simulink model "Purdue_Sim"  (R2018b)
settings: Solver=VariableStepAuto  StartTime=0.0  StopTime=300  FixedStep=0.0001  RelTol=1e-7
values from neighbouring files (symbols this model uses):
  alpha_data = load('alpha_data.csv')    [One_Run.m]    (also in Test_Runs_Arthur_Function.m; eqns_motion_script.m; eqns_motion_script_439.m)
  AR = De^2/Dt^2    (= 7.35623218146)    [One_Run.m]    (also in Test_Runs_Arthur_Function.m; engineMass.m = engine.output.eql.aeat(3); eqns_motion_script_439.m = 7.52170654272)
  At = pi*Dt^2/4    (= 7.87496924005)    [One_Run.m]    (also in Test_Runs_Arthur_Function.m; engineMass.m = cstar*mdot/(Pc*g); eqns_motion_script_439.m = 7.53210209316)
  burn_time = (200000+Impulse_Savings)/Thrust    (= 39.2156862745)    [One_Run.m]    (also in Purdue_Setup.m = 40; Setup.m = 42; Test_Runs.m = 40; Test_Runs_Arthur_Function.m = 42.7553241067)
  Cd_data = load('cd_M.csv')    [One_Run.m]    (also in Test_Runs_Arthur_Function.m; eqns_motion_script.m; eqns_motion_script_439.m)
  Cn_data = load('cl_M_a.csv')    [One_Run.m]    (also in Test_Runs_Arthur_Function.m; eqns_motion_script.m; eqns_motion_script_439.m)
  Cp_data = load('cp_M_a.csv')    [One_Run.m]    (also in Test_Runs_Arthur_Function.m; eqns_motion_script.m; eqns_motion_script_439.m)
  De = 8.5883    [One_Run.m]    (also in Test_Runs_Arthur_Function.m; engineMass.m = sqrt(4*Ae/pi); eqns_motion_script_439.m = 8.4932)
  diameter_ft = diameter/12    (= 1.5)    [One_Run.m]    (also in Purdue_Setup.m; Setup.m = 0.535416666667; Test_Runs.m; Test_Runs_Arthur_Function.m)
  dry_mass_slugs = dry_mass / 32.2    (= 16.4109852637)    [One_Run.m]    (also in Purdue_Setup.m = 12.4223602484; Setup.m = 1.28260869565; Test_Runs.m = dry_mass / 32.2; Test_Runs_Arthur_Function.m = dry_mass / 32.2)
  initial_height = 4595    [One_Run.m]    (also in Purdue_Setup.m = 4600; Setup.m = 0; Test_Runs.m = 0; Test_Runs_Arthur_Function.m)
  latitude = 32.9861    [One_Run.m]    (also in Test_Runs_Arthur_Function.m)
  longitude = -106.9717    [One_Run.m]    (also in Test_Runs_Arthur_Function.m)
  M_data = load('M_data.csv')    [One_Run.m]    (also in Test_Runs_Arthur_Function.m; eqns_motion_script.m; eqns_motion_script_439.m)
  m_dot_slugs = m_dot / 32.2    (= 0.725155279503)    [One_Run.m]    (also in Purdue_Setup.m = -0.621118012422; Setup.m = 0.0567139899438; Test_Runs.m = -0.621118012422; Test_Runs_Arthur_Function.m = -0.62217941157)
  mass_inert = 523.36 + margin    (= 523.36)    [One_Run.m]    (also in Setup.m = 41.3; Test_Runs.m = mass_engine + mass_pump + tank(1).mass +tank(2).mass + mass_; Test_Runs_Arthur_Function.m = mass_engine + mass_pump + tank(1).mass +tank(2).mass + inter)
  Pc = 450    [One_Run.m]    (also in Test_Runs_Arthur_Function.m; eqns_motion_script_439.m)
  Pe = 10    [One_Run.m]    (also in Test_Runs.m = pressure_integral(end)/burn_time; Test_Runs_Arthur_Function.m; eqns_motion_script_439.m)
  rocket_length = 24    [One_Run.m]    (also in Setup.m; Test_Runs.m; Test_Runs_Arthur_Function.m)
  Throttle_end_time = 35    [One_Run.m]    (also in Setup.m; Test_Runs.m = 0; Test_Runs_Arthur_Function.m = 0)
  Throttle_start_time = 15    [One_Run.m]    (also in Setup.m; Test_Runs.m = 0; Test_Runs_Arthur_Function.m = 0)
  Throttled_m_dot = m_dot_slugs*(1 - throttle)    (= 0.725155279503)    [One_Run.m]    (also in Setup.m = 0.0567139899438; Test_Runs.m = -0.621118012422; Test_Runs_Arthur_Function.m = -0.62217941157)
  Thrust = 5100    [One_Run.m]    (also in Purdue_Setup.m = 5000; Setup.m = 800; Test_Runs.m = 5000; Test_Runs_Arthur_Function.m = 4677.78)
  wet_mass_slugs = wet_mass / 32.2    (= 44.848447205)    [One_Run.m]    (also in Purdue_Setup.m = 37.2670807453; Setup.m = 3.66459627329; Test_Runs.m = wet_mass / 32.2; Test_Runs_Arthur_Function.m = wet_mass / 32.2)
libraries: vrlib x8, aerolibconvert2 x5, aerolibasang x3, simulink_extras x3, aerolibutil x2, simulink x2, aerolibanimutils x2, shared6dof x1, sharedutil x1, aerolibadyn x1, aerolibatmos2 x1, aerolibtransform2 x1
settings Model: Creator=jbartkie  LastModifiedBy=bartk
settings DataIOCC: ExternalInput=getinputstruct(op_snapshot1)  InitialState=getstatestruct(op_snapshot1)
settings DebuggingCC: LibraryContextMissingDiagnostic=none
settings SFSimCC: SimUseLocalCustomCode=off
settings RTWCC: RTWUseLocalCustomCode=off

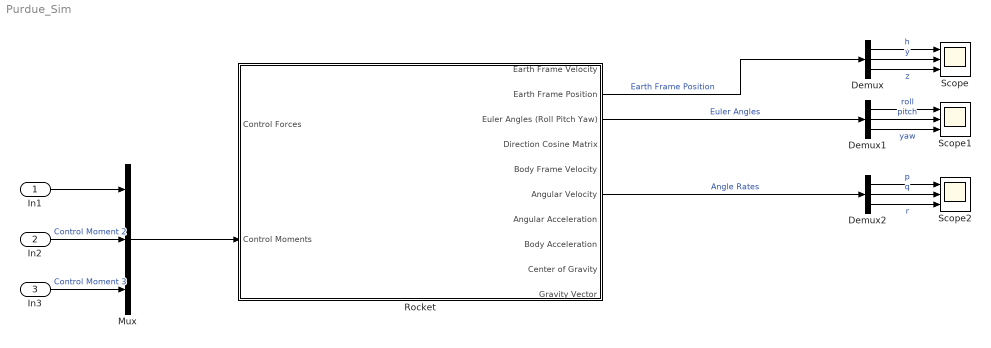
== system Purdue_Sim ==
  In1 : Inport
  In2 : Inport  Port=2
  In3 : Inport  Port=3
  Demux : Demux  Outputs=3
  Demux1 : Demux  Outputs=3
  Demux2 : Demux  Outputs=3
  Mux : Mux  Inputs=3
  Rocket : Subsystem
  Scope : Scope  NumInputPorts=3
  Scope1 : Scope  NumInputPorts=3
  Scope2 : Scope  NumInputPorts=3
  wires:
  Mux/1 -> Rocket/2(Control Moments)
  In2/1 -> Mux/2  "Control Moment 2"
  In3/1 -> Mux/3  "Control Moment 3"
  Rocket/6(Angular Velocity) -> Demux2/1  "Angle Rates"
  Rocket/3(Euler Angles (Roll Pitch Yaw)) -> Demux1/1  "Euler Angles"
  Rocket/2(Earth Frame Position) -> Demux/1  "Earth Frame Position"
  Demux/1 -> Scope/1  "h"
  Demux/2 -> Scope/2  "y"
  Demux/3 -> Scope/3  "z"
  Demux1/1 -> Scope1/1  "roll"
  Demux1/2 -> Scope1/2  "pitch"
  Demux1/3 -> Scope1/3  "yaw"
  Demux2/1 -> Scope2/1  "p"
  Demux2/2 -> Scope2/2  "q"
  Demux2/3 -> Scope2/3  "r"
  In1/1 -> Mux/1

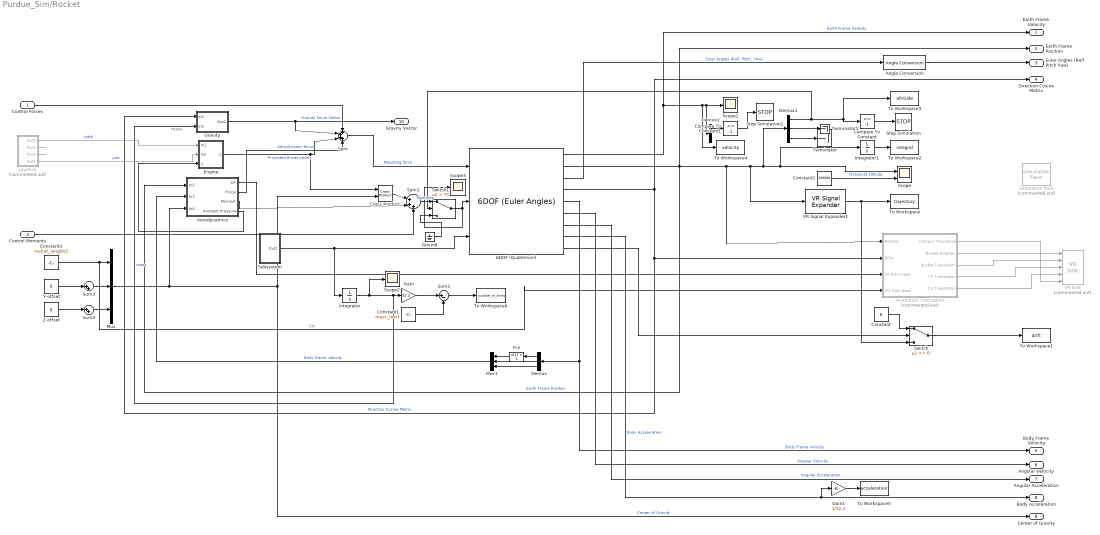
== system Purdue_Sim/Rocket ==
  note: mass
  Control Forces : Inport
  Control Moments : Inport  Port=2
  6DOF (Quaternion) : shared6dof/6DOF (Euler Angles)  units=English (Velocity in ft/s)  mtype=Simple Variable  rep=Quaternion  xme_0=[initial_height 0 0]  Vm_0=[0 0 0]  eul_0=[0 0*pi/180 0]  pm_0=[0 0 0]  mass_0=wet_mass_slugs  mass_e=dry_mass_slugs  mass_f=wet_mass_slugs  inertia=eye(3)  inertia_e=I_wet  inertia_f=I_dry  k_quat=1.0  vre_flag=off  abi_flag=off  aMode=0  xme_statename=''  Vm_statename=''  eul_statename=''  quat_statename=''  pm_statename=''  mass_statename=''
      settings: SourceProductBaseCode=AE
  "Aerodynamics " : Subsystem
  Angle Conversion : aerolibconvert2/Angle Conversion  IU=rad  OU=deg
  Animation Translation : Subsystem  Commented=on
  Compare To Constant : simulink/Logic and Bit Operations/Compare To Constant  relop=<=  const=-1  OutDataTypeStr=boolean
  Compare To Constant1 : simulink/Logic and Bit Operations/Compare To Constant  relop=<=  const=-1  OutDataTypeStr=boolean
  Constant : Constant  Value=0
  Constant1 : Constant  Value=mass_inert
  Constant2 : Constant  Value=328084
  Constant3 : Constant  Value=rocket_length/2
  Cross Product : vrlib/Utilities/Cross Product
      settings: SourceProductBaseCode=VR
  Demux : Demux  Outputs=3
  Demux1 : Demux  Outputs=3
  Demux2 : Demux  Outputs=3
  "Engine " : Subsystem
  Fcn : Fcn  Expr=u(1) + 1
  Gain : Gain  Gain=32.2
  Gain1 : Gain  Gain=1/32.2
  Gravity : Subsystem
  Ground : Ground
  Integrator : Integrator  InitialCondition=wet_mass_slugs  LimitOutput=on  LowerSaturationLimit=dry_mass_slugs
  Integrator1 : Integrator
  Joystick : Subsystem  Commented=on
  Mux : Mux  Inputs=3
  Mux1 : Mux  Inputs=3
  Scope : Scope  NumInputPorts=2
  Scope1 : Scope
  Scope2 : Scope
  Scope3 : Scope
  Simulation Pace : aerolibanimutils/Simulation Pace  Commented=on  SimulationPace=1  SleepMode=MATLAB Thread  OutputPaceError=off  SampleTime=1/30
  Stop Simulation : Stop
  Stop Simulation1 : Stop
  Subsystem : Subsystem
  Sum : Sum  Inputs=++++
  Sum1 : Sum  Inputs=|+++
  Sum2 : Sum  Inputs=|+-
  Sum3 : Sum  Inputs=|++
  Sum4 : Sum  Inputs=|++
  Switch : Switch
  Switch1 : Switch  Criteria=u2 > Threshold  Threshold=75
  Terminator : Terminator
  Terminator1 : Terminator
  To Workspace : ToWorkspace  VariableName=trajectory  SampleTime=-1
  To Workspace1 : ToWorkspace  VariableName=drift  SampleTime=-1
  To Workspace2 : ToWorkspace  VariableName=integral  SampleTime=-1
  To Workspace3 : ToWorkspace  VariableName=altitude  SampleTime=-1
  To Workspace4 : ToWorkspace  VariableName=velocity  SampleTime=-1
  To Workspace5 : ToWorkspace  VariableName=acceleration  SampleTime=-1
  To Workspace6 : ToWorkspace  VariableName=oxidizer_m_array  SampleTime=-1
  VR Signal Expander1 : vrlib/VR Signal Expander  outwidth=3  outidx=[3 2 1]
      settings: SourceProductName=Simulink 3D Animation  SourceProductBaseCode=VR
  VR Sink : vrlib/VR Sink  Commented=on  InstantiateOnLoad=on  SampleTime=0.1  ViewEnable=on  RemoteChange=off  RemoteView=off  FieldsWritten=Rocket.rotation.4.1.1.double#Rocket.translation.3.1.1.double#CP.translation.3.1.1.double#CG.translation.3.1.1.double#Camera.position.3.1.1.double  WorldFileName=liftoff.WRL  AutoView=off  VideoDimensions=[]  AllowVariableSize=off
      settings: SourceProductBaseCode=VR
  Y-offset : Constant  Value=0
  Z-offset : Constant  Value=0
  Earth Frame Velocity : Outport
  Earth Frame Position : Outport  Port=2
  Euler Angles (Roll Pitch Yaw) : Outport  Port=3
  Direction Cosine Matrix : Outport  Port=4
  Body Frame Velocity : Outport  Port=5
  Angular Velocity : Outport  Port=6
  Angular Acceleration : Outport  Port=7
  Body Acceleration : Outport  Port=8
  Center of Gravity : Outport  Port=9
  Gravity Vector : Outport  Port=10
  wires:
  Demux/3 -> Mux1/3
  6DOF (Quaternion)/4 -> Gravity/1(In1), Animation Translation/2(DCM), Direction Cosine Matrix/1  "Direction Cosine Matrix"
  6DOF (Quaternion)/2 -> VR Signal Expander1/1, Demux1/1, Integrator1/1, Scope/1, Animation Translation/1(Position), "Aerodynamics "/1(In2), Earth Frame Position/1  "Earth Frame Position"
  6DOF (Quaternion)/1 -> Earth Frame Velocity/1, To Workspace4/1, Demux2/1, Scope1/1  "Earth Frame Velocity"
  6DOF (Quaternion)/3 -> Angle Conversion/1  "Euler Angles (Roll, Pitch, YAw)"
  6DOF (Quaternion)/7 -> Angular Acceleration/1  "Angular Acceleration"
  6DOF (Quaternion)/8 -> Gain1/1, Body Acceleration/1  "Body Acceleration"
  Mux/1 -> Cross Product/2, Center of Gravity/1, "Aerodynamics "/3(In4)  "Center of Gravity"
  6DOF (Quaternion)/6 -> Angular Velocity/1  "Angular Velocity"
  Cross Product/1 -> Sum1/1
  Gravity/1(Out1) -> Gravity Vector/1, Sum/2  "Gravity Force Vector"
  6DOF (Quaternion)/5 -> Demux/1, Body Frame Velocity/1  "Body Frame Velocity"
  Control Moments/1 -> Sum1/3
  Control Forces/1 -> Sum/1
  Integrator/1 -> Scope2/1, Gravity/2(In2), Gain/1  "mass"
  Sum/1 -> 6DOF (Quaternion)/1  "Resulting force"
  Joystick/1(Out1) -> "Engine "/1(In1)  "pitch"
  "Engine "/1(Out1) -> Cross Product/1, Sum/3  "Projected thrust vector"
  Demux1/3 -> Terminator/1
  Joystick/4(Out4) -> "Engine "/2(In2)  "yaw"
  Switch/1 -> To Workspace1/1
  Demux/2 -> Mux1/2
  Demux/1 -> Fcn/1
  Fcn/1 -> Mux1/1
  Mux1/1 -> "Aerodynamics "/2(In3)  "Body frame velocity"
  VR Signal Expander1/1 -> Switch/3, To Workspace/1
  "Aerodynamics "/1(CP) -> Animation Translation/3(CP from base)
  Constant/1 -> Switch/1
  Joystick/2(Out2) -> ?
  Compare To Constant/1 -> Stop Simulation/1
  Integrator1/1 -> To Workspace2/1
  Joystick/3(Out3) -> ?
  Demux1/2 -> Terminator1/1
  Demux1/1 -> Switch1/2, Compare To Constant/1, To Workspace3/1
  6DOF (Quaternion)/9 -> Switch/2
  Constant3/1 -> Mux/1, Animation Translation/4(CG from base)  "CG"
  Animation Translation/2(Rocket Rotation) -> VR Sink/1
  Animation Translation/3(Rocket Translation) -> VR Sink/2
  Animation Translation/4(CP Translation) -> VR Sink/3
  Animation Translation/5(CG Translation) -> VR Sink/4
  Animation Translation/1(Camera Translation) -> VR Sink/5
  Constant2/1 -> Scope/2  "threshold altitude"
  Angle Conversion/1 -> Euler Angles (Roll Pitch Yaw)/1
  "Aerodynamics "/3(Moment) -> Sum1/2
  "Aerodynamics "/2(Force) -> Sum/4  "Aerodynamic force"
  Constant1/1 -> Sum2/2
  Gain/1 -> Sum2/1
  Sum2/1 -> To Workspace6/1
  Compare To Constant1/1 -> Stop Simulation1/1
  Y-offset/1 -> Sum3/1
  Sum3/1 -> Mux/2
  Z-offset/1 -> Sum4/1
  Sum4/1 -> Mux/3
  Demux2/1 -> Compare To Constant1/1
  Subsystem/1(Out1) -> 6DOF (Quaternion)/3, Integrator/1
  Gain1/1 -> To Workspace5/1
  "Aerodynamics "/4(Ambient Pressure) -> "Engine "/3(Ambient Pressure)
  Sum1/1 -> Switch1/1  "Moments"
  Switch1/1 -> 6DOF (Quaternion)/2, Scope3/1
  Ground/1 -> Switch1/3

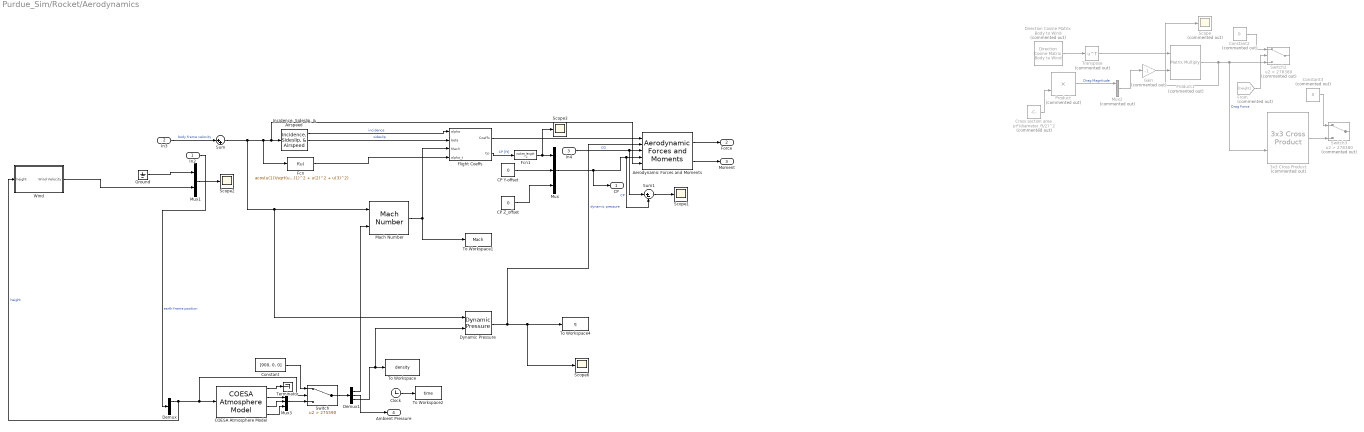
== system Purdue_Sim/Rocket/Aerodynamics  ==
  In2 : Inport
  In3 : Inport  Port=2
  In4 : Inport  Port=3
  3x3 Cross Product : sharedutil/3x3 Cross Product  Commented=on  aMode=aMode
      settings: SourceProductBaseCode=AE
  "Aerodynamic Forces and Moments " : aerolibadyn/Aerodynamic Forces and Moments   inputAxes=Wind  outputForceAxes=Body  outputMomentAxes=Body  S=S  b=diameter_ft  cbar=rocket_length
      settings: SourceProductName=Aerospace Blockset
  COESA Atmosphere Model : aerolibatmos2/COESA Atmosphere Model  units=English (Velocity in ft/s)  spec=1976 COESA-extended U.S. Standard Atmosphere  model=Profile  profile_var=High temperature  profile_percent=1%  profile_alt=5 km (16404 ft)  envelope_var=High temperature  envelope_percent=1%  action=Warning
  "CP Y-offset " : Constant  Value=0
  "CP Z_offset " : Constant  Value=0
  Clock : Clock
  Constant : Constant  Value=[900, 0, 0]
  Constant2 : Constant  Commented=on  Value=0
  Constant3 : Constant  Commented=on  Value=0
  Cross section area : Constant  Commented=on  Value=pi*(diameter_ft/2)^2  VectorParams1D=off
  Demux : Demux  Outputs=3
  Demux1 : Demux  Outputs=3
  Direction Cosine Matrix Body to Wind : aerolibtransform2/Direction Cosine Matrix Body to Wind  Commented=on
      settings: SourceProductName=Aerospace Blockset  SourceProductBaseCode=AE
  Dynamic Pressure : aerolibasang/Dynamic Pressure
  Fcn : Fcn  Expr=acos(u(1))/sqrt(u(1)^2 + u(2)^2 + u(3)^2)
  Fcn1 : Fcn  Expr=rocket_length - u
  Flight Coeffs : Subsystem
  From : From  Commented=on  GotoTag=height
  Gain : Gain  Commented=on  Gain=-1
  Ground : Ground
  "Incidence, Sideslip, & Airspeed" : aerolibasang/Incidence, Sideslip, & Airspeed
      settings: SourceProductName=Aerospace Blockset
  Mach Number : aerolibasang/Mach Number
      settings: SourceProductName=Aerospace Blockset  SourceProductBaseCode=AE
  Mux : Mux  Inputs=3
  Mux1 : Mux  Inputs=2
  Mux2 : Mux  Commented=on  Inputs=3
  Mux3 : Mux  Inputs=3
  Product : Product  Commented=on  Inputs=3
  Product1 : Product  Commented=on  Multiplication=Matrix(*)
  Scope : Scope  Commented=on
  Scope{1..3,6} (4 alike) : Scope
  Sum : Sum  Inputs=|++
  Sum1 : Sum  Inputs=|+-
  Switch : Switch  Criteria=u2 > Threshold  Threshold=275590
  Switch2 : Switch  Commented=on  Criteria=u2 > Threshold  Threshold=278380
  Switch3 : Switch  Commented=on  Criteria=u2 > Threshold  Threshold=278380
  Terminator : Terminator
  To Workspace : ToWorkspace  VariableName=density  SampleTime=-1
  To Workspace1 : ToWorkspace  VariableName=Mach  SampleTime=-1
  To Workspace2 : ToWorkspace  VariableName=time  SampleTime=-1
  To Workspace4 : ToWorkspace  VariableName=q  SaveFormat=Timeseries  SampleTime=-1
  Transpose : Math  Commented=on  Operator=transpose  SaturateOnIntegerOverflow=on
  Wind : Subsystem
  CP : Outport
  Force : Outport  Port=2
  Moment : Outport  Port=3
  Ambient Pressure : Outport  Port=4
  wires:
  In2/1 -> Demux/1  "earth frame position"
  "Incidence, Sideslip, & Airspeed"/1 -> Flight Coeffs/1(alpha)  "incidence"
  "Incidence, Sideslip, & Airspeed"/2 -> Flight Coeffs/2(beta)  "sideslip"
  Mach Number/1 -> To Workspace1/1, Flight Coeffs/3(Mach)
  "CP Y-offset "/1 -> Mux/2
  "CP Z_offset "/1 -> Mux/3
  Flight Coeffs/2(Cp) -> Fcn1/1  "CP [ft]"
  Clock/1 -> To Workspace2/1
  Dynamic Pressure/1 -> "Aerodynamic Forces and Moments "/2, Scope6/1, To Workspace4/1  "dynamic pressure"
  Demux/1 -> Wind/1(height), Switch/2, COESA Atmosphere Model/1  "height"
  Flight Coeffs/1(Coeffs) -> "Aerodynamic Forces and Moments "/1
  Transpose/1 -> Product1/1
  Direction Cosine Matrix Body to Wind/1 -> Transpose/1
  Product/1 -> Mux2/1  "Drag Magnitude"
  From/1 -> Switch2/2
  ? -> 3x3 Cross Product/1
  Constant2/1 -> Switch2/1
  Gain/1 -> Product1/2
  ? -> Product/1
  Constant3/1 -> Switch3/1
  3x3 Cross Product/1 -> Switch3/3
  Mux2/1 -> Gain/1
  ? -> Product/2  "dynamic pressure"
  ? -> Direction Cosine Matrix Body to Wind/1
  Cross section area/1 -> Product/3
  Product1/1 -> Scope/1, Switch2/3, 3x3 Cross Product/2  "Drag Force"
  Mux/1 -> Sum1/2, "Aerodynamic Forces and Moments "/4, CP/1  "CP"
  "Aerodynamic Forces and Moments "/1 -> Force/1
  "Aerodynamic Forces and Moments "/2 -> Moment/1
  Fcn/1 -> Flight Coeffs/4(alpha_t)
  In3/1 -> Sum/1  "body frame velocity"
  Sum/1 -> Dynamic Pressure/1, Mach Number/1, Fcn/1, "Aerodynamic Forces and Moments "/5, "Incidence, Sideslip, & Airspeed"/1
  Sum1/1 -> Scope1/1
  Fcn1/1 -> Scope3/1, Mux/1
  In4/1 -> Sum1/1, "Aerodynamic Forces and Moments "/3  "CG"
  Wind/1(Wind Velocity) -> Mux1/2
  Ground/1 -> Mux1/1
  Mux1/1 -> Scope2/1
  COESA Atmosphere Model/1 -> Terminator/1
  COESA Atmosphere Model/2 -> Mux3/1
  COESA Atmosphere Model/3 -> Mux3/2
  COESA Atmosphere Model/4 -> Mux3/3
  Mux3/1 -> Switch/3
  Constant/1 -> Switch/1
  Switch/1 -> Demux1/1
  Demux1/3 -> Dynamic Pressure/2, To Workspace/1
  Demux1/1 -> Mach Number/2
  Demux1/2 -> Ambient Pressure/1

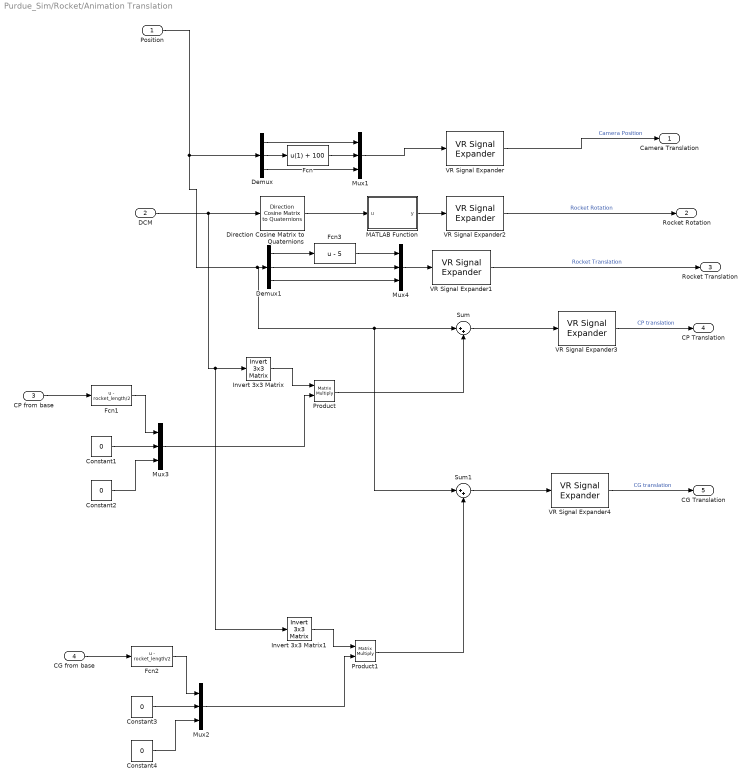
== system Purdue_Sim/Rocket/Animation Translation ==
  Position : Inport
  DCM : Inport  Port=2
  CP from base : Inport  Port=3
  CG from base : Inport  Port=4
  Constant{1..4} (4 alike) : Constant  Value=0
  Demux : Demux  Outputs=3
  Demux1 : Demux  Outputs=3
  Direction Cosine Matrix to Quaternions : sharedtransform/Direction Cosine Matrix  to Quaternions  aMode=0  action=None  tolerance=eps(2)
      settings: SourceProductName=Aerospace Blockset  SourceProductBaseCode=AE
  Fcn : Fcn  Expr=u(1) + 100
  Fcn1 : Fcn  Expr=u - rocket_length/2
  Fcn2 : Fcn  Expr=u - rocket_length/2
  Fcn3 : Fcn  Expr=u - 5
  Invert 3x3 Matrix : aerolibutil/Invert  3x3 Matrix
  Invert 3x3 Matrix1 : aerolibutil/Invert  3x3 Matrix
  MATLAB Function : MATLAB Function  TreatAsAtomicUnit=on
  Mux{1..4} (4 alike) : Mux  Inputs=3
  Product : Product  Multiplication=Matrix(*)
  Product1 : Product  Multiplication=Matrix(*)
  Sum : Sum  Inputs=|++
  Sum1 : Sum  Inputs=|++
  VR Signal Expander{,1,3..4} (4 alike) : vrlib/VR Signal Expander  outwidth=3  outidx=[2 3 1]
      settings: SourceProductName=Simulink 3D Animation  SourceProductBaseCode=VR
  VR Signal Expander2 : vrlib/VR Signal Expander  outwidth=4  outidx=[2 3 1 4]
      settings: SourceProductName=Simulink 3D Animation  SourceProductBaseCode=VR
  Camera Translation : Outport
  Rocket Rotation : Outport  Port=2
  Rocket Translation : Outport  Port=3
  CP Translation : Outport  Port=4
  CG Translation : Outport  Port=5
  wires:
  Demux/2 -> Fcn/1
  Position/1 -> Demux1/1, Sum1/1, Sum/1, Demux/1
  Mux1/1 -> VR Signal Expander/1
  MATLAB Function/1(y) -> VR Signal Expander2/1
  DCM/1 -> Invert 3x3 Matrix1/1, Invert 3x3 Matrix/1, Direction Cosine Matrix to Quaternions/1
  Direction Cosine Matrix to Quaternions/1 -> MATLAB Function/1(u)
  Demux/3 -> Mux1/3
  Demux/1 -> Mux1/1
  Fcn/1 -> Mux1/2
  VR Signal Expander/1 -> Camera Translation/1  "Camera Position"
  CP from base/1 -> Fcn1/1
  VR Signal Expander3/1 -> CP Translation/1  "CP translation"
  Constant1/1 -> Mux3/2
  Fcn1/1 -> Mux3/1
  Constant2/1 -> Mux3/3
  Mux3/1 -> Product/2
  Product/1 -> Sum/2
  Invert 3x3 Matrix/1 -> Product/1
  Sum/1 -> VR Signal Expander3/1
  VR Signal Expander2/1 -> Rocket Rotation/1  "Rocket Rotation"
  VR Signal Expander1/1 -> Rocket Translation/1  "Rocket Translation"
  Constant4/1 -> Mux2/3
  Invert 3x3 Matrix1/1 -> Product1/1
  Mux2/1 -> Product1/2
  Fcn2/1 -> Mux2/1
  Constant3/1 -> Mux2/2
  CG from base/1 -> Fcn2/1
  Product1/1 -> Sum1/2
  Sum1/1 -> VR Signal Expander4/1
  VR Signal Expander4/1 -> CG Translation/1  "CG translation"
  Demux1/3 -> Mux4/3
  Demux1/2 -> Mux4/2
  Mux4/1 -> VR Signal Expander1/1
  Demux1/1 -> Fcn3/1
  Fcn3/1 -> Mux4/1

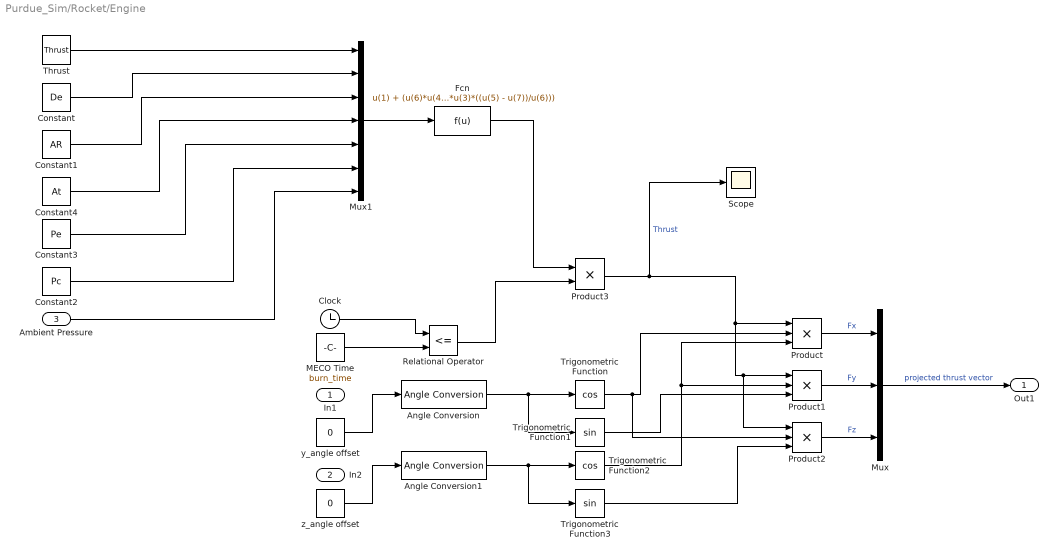
== system Purdue_Sim/Rocket/Engine  ==
  In1 : Inport
  In2 : Inport  Port=2
  Ambient Pressure : Inport  Port=3
  Angle Conversion : aerolibconvert2/Angle Conversion  IU=deg  OU=rad
  Angle Conversion1 : aerolibconvert2/Angle Conversion  IU=deg  OU=rad
  Clock : Clock
  Constant : Constant  Value=De
  Constant1 : Constant  Value=AR
  Constant2 : Constant  Value=Pc
  Constant3 : Constant  Value=Pe
  Constant4 : Constant  Value=At
  Fcn : Fcn  Expr=u(1) + (u(6)*u(4)*u(3)*((u(5) - u(7))/u(6)))
  MECO Time : Constant  Value=burn_time
  Mux : Mux  Inputs=3
  Mux1 : Mux  Inputs=7
  Product : Product  Inputs=3
  Product1 : Product  Inputs=3
  Product2 : Product  Inputs=3
  Product3 : Product
  Relational Operator : RelationalOperator  Operator=<=  OutDataTypeStr=boolean  RndMeth=Simplest
  Scope : Scope
  Thrust : Constant  Value=Thrust
  Trigonometric Function : Trigonometry  Operator=cos
  Trigonometric Function1 : Trigonometry
  Trigonometric Function2 : Trigonometry  Operator=cos
  Trigonometric Function3 : Trigonometry
  y_angle offset : Constant  Value=0
  z_angle offset : Constant  Value=0
  Out1 : Outport
  wires:
  Angle Conversion/1 -> Trigonometric Function1/1, Trigonometric Function/1
  Angle Conversion1/1 -> Trigonometric Function3/1, Trigonometric Function2/1
  Clock/1 -> Relational Operator/1
  MECO Time/1 -> Relational Operator/2
  Relational Operator/1 -> Product3/2
  Product/1 -> Mux/1  "Fx"
  Product1/1 -> Mux/2  "Fy"
  Product2/1 -> Mux/3  "Fz"
  Mux/1 -> Out1/1  "projected thrust vector"
  Product3/1 -> Scope/1, Product2/1, Product1/1, Product/1  "Thrust"
  Trigonometric Function2/1 -> Product1/2, Product/3
  Trigonometric Function/1 -> Product2/2, Product/2
  Trigonometric Function1/1 -> Product1/3
  Trigonometric Function3/1 -> Product2/3
  y_angle offset/1 -> Angle Conversion/1
  z_angle offset/1 -> Angle Conversion1/1
  Thrust/1 -> Mux1/1
  Constant/1 -> Mux1/2
  Constant1/1 -> Mux1/3
  Constant4/1 -> Mux1/4
  Constant3/1 -> Mux1/5
  Constant2/1 -> Mux1/6
  Ambient Pressure/1 -> Mux1/7
  Mux1/1 -> Fcn/1
  Fcn/1 -> Product3/1

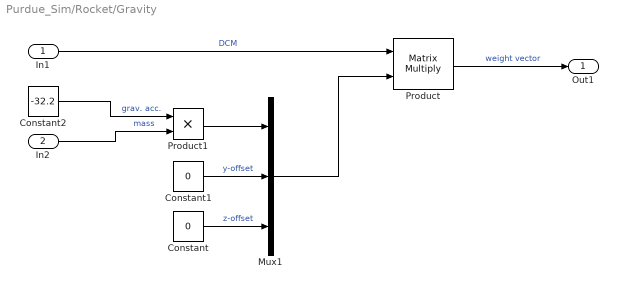
== system Purdue_Sim/Rocket/Gravity ==
  In1 : Inport
  In2 : Inport  Port=2
  Constant : Constant  Value=0
  Constant1 : Constant  Value=0
  Constant2 : Constant  Value=-32.2
  Mux1 : Mux  Inputs=3
  Product : Product  Multiplication=Matrix(*)
  Product1 : Product
  Out1 : Outport
  wires:
  Mux1/1 -> Product/2
  Product/1 -> Out1/1  "weight vector"
  In1/1 -> Product/1  "DCM"
  Constant1/1 -> Mux1/2  "y-offset"
  Constant2/1 -> Product1/1  "grav. acc."
  In2/1 -> Product1/2  "mass"
  Product1/1 -> Mux1/1
  Constant/1 -> Mux1/3  "z-offset"

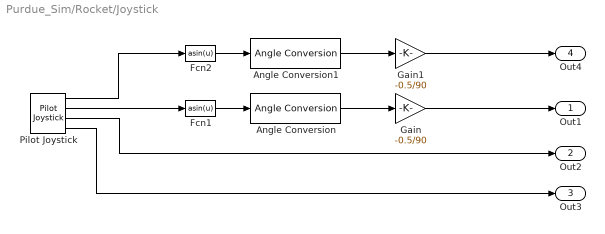
== system Purdue_Sim/Rocket/Joystick ==
  Angle Conversion : aerolibconvert2/Angle Conversion  IU=rad  OU=deg
  Angle Conversion1 : aerolibconvert2/Angle Conversion  IU=rad  OU=deg
  Fcn1 : Fcn  Expr=asin(u)
  Fcn2 : Fcn  Expr=asin(u)
  Gain : Gain  Gain=-0.5/90
  Gain1 : Gain  Gain=-0.5/90
  Pilot Joystick : aerolibanimutils/Pilot Joystick  JoystickID=Joystick1  OutputConfiguration=FourAxis  SampleTime=1/30
  Out1 : Outport
  Out2 : Outport  Port=2
  Out3 : Outport  Port=3
  Out4 : Outport  Port=4
  wires:
  Angle Conversion/1 -> Gain/1
  Fcn2/1 -> Angle Conversion1/1
  Gain1/1 -> Out4/1
  Angle Conversion1/1 -> Gain1/1
  Pilot Joystick/3 -> Out2/1
  Fcn1/1 -> Angle Conversion/1
  Pilot Joystick/2 -> Fcn1/1
  Pilot Joystick/1 -> Fcn2/1
  Gain/1 -> Out1/1
  Pilot Joystick/4 -> Out3/1

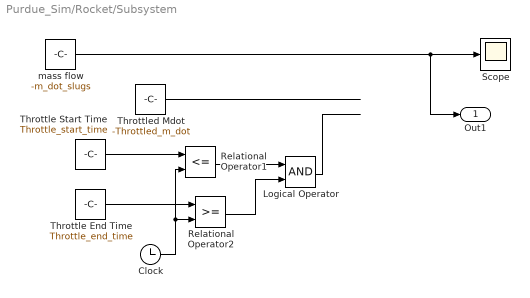
== system Purdue_Sim/Rocket/Subsystem ==
  Clock : Clock
  Logical Operator : Logic  AllPortsSameDT=off  OutDataTypeStr=boolean
  Relational Operator1 : RelationalOperator  Operator=<=  OutDataTypeStr=boolean  RndMeth=Simplest
  Relational Operator2 : RelationalOperator  OutDataTypeStr=boolean  RndMeth=Simplest
  Scope : Scope
  Throttle End Time : Constant  Value=Throttle_end_time
  Throttle Start Time : Constant  Value=Throttle_start_time
  Throttled Mdot : Constant  Value=-Throttled_m_dot
  mass flow : Constant  Value=-m_dot_slugs
  Out1 : Outport
  wires:
  Clock/1 -> Relational Operator1/2, Relational Operator2/2
  Relational Operator1/1 -> Logical Operator/1
  Throttled Mdot/1 -> ?
  Relational Operator2/1 -> Logical Operator/2
  mass flow/1 -> Out1/1, Scope/1
  Throttle Start Time/1 -> Relational Operator1/1
  Throttle End Time/1 -> Relational Operator2/1
  Logical Operator/1 -> ?

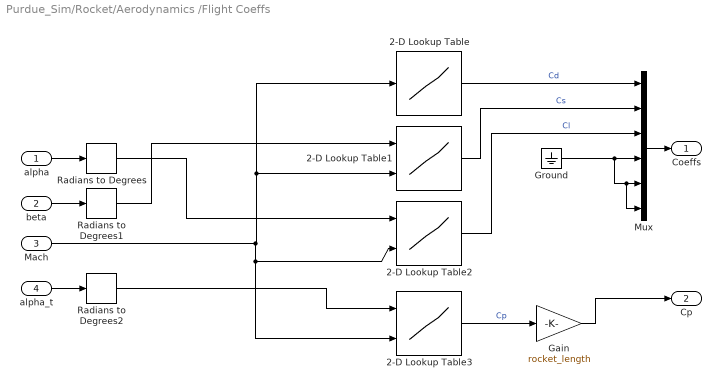
== system Purdue_Sim/Rocket/Aerodynamics /Flight Coeffs ==
  alpha : Inport
  beta : Inport  Port=2
  Mach : Inport  Port=3
  alpha_t : Inport  Port=4
  2-D Lookup Table : Lookup_n-D  NumberOfTableDimensions=1  BreakpointsForDimension1=M_data  BreakpointsForDimension2=[1:3]  Table=Cd_data  InternalRulePriority=Speed  RndMeth=Simplest  InputSameDT=on
  2-D Lookup Table1 : Lookup_n-D  BreakpointsForDimension1=alpha_data  BreakpointsForDimension2=M_data  Table=Cn_data  InternalRulePriority=Speed  RndMeth=Simplest  InputSameDT=on
  2-D Lookup Table2 : Lookup_n-D  BreakpointsForDimension1=alpha_data  BreakpointsForDimension2=M_data  Table=Cn_data  InternalRulePriority=Speed  RndMeth=Simplest  InputSameDT=on
  2-D Lookup Table3 : Lookup_n-D  BreakpointsForDimension1=alpha_data  BreakpointsForDimension2=M_data  Table=Cp_data  InternalRulePriority=Speed  RndMeth=Simplest  InputSameDT=on
  Gain : Gain  Gain=rocket_length
  Ground : Ground
  Mux : Mux  Inputs=6
  Radians to Degrees : simulink_extras/Transformations/Radians to Degrees
  Radians to Degrees1 : simulink_extras/Transformations/Radians to Degrees
  Radians to Degrees2 : simulink_extras/Transformations/Radians to Degrees
  Coeffs : Outport
  Cp : Outport  Port=2
  wires:
  alpha/1 -> Radians to Degrees/1
  beta/1 -> Radians to Degrees1/1
  alpha_t/1 -> Radians to Degrees2/1
  2-D Lookup Table/1 -> Mux/1  "Cd"
  Mux/1 -> Coeffs/1
  2-D Lookup Table1/1 -> Mux/2  "Cs"
  2-D Lookup Table2/1 -> Mux/3  "Cl"
  Ground/1 -> Mux/6, Mux/5, Mux/4
  Mach/1 -> 2-D Lookup Table3/2, 2-D Lookup Table2/2, 2-D Lookup Table/1, 2-D Lookup Table1/2
  Radians to Degrees/1 -> 2-D Lookup Table2/1
  Radians to Degrees1/1 -> 2-D Lookup Table1/1
  Radians to Degrees2/1 -> 2-D Lookup Table3/1
  2-D Lookup Table3/1 -> Gain/1  "Cp"
  Gain/1 -> Cp/1

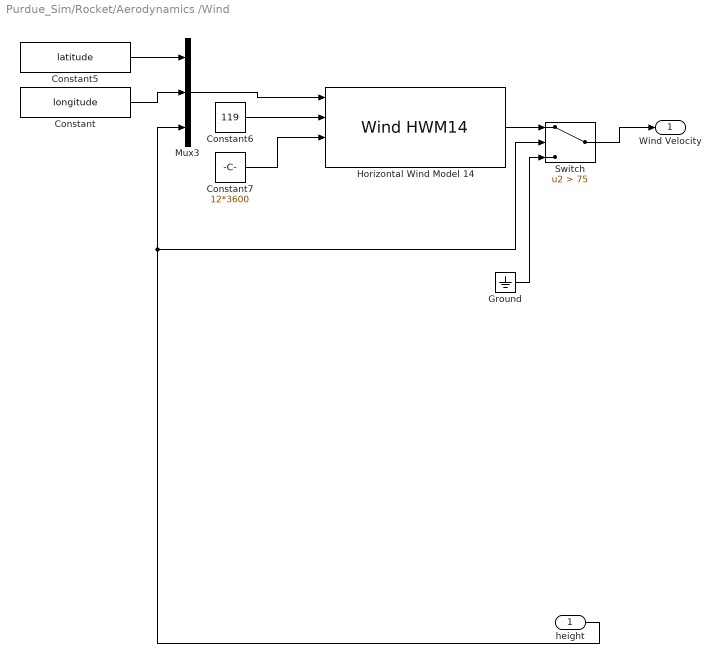
== system Purdue_Sim/Rocket/Aerodynamics /Wind ==
  height : Inport
  Constant : Constant  Value=longitude
  Constant5 : Constant  Value=latitude
  Constant6 : Constant  Value=119
  Constant7 : Constant  Value=12*3600
  Ground : Ground
  Horizontal Wind Model 14 : WindHWM14  units=English (Velocity in ft/s)  model=Total
  Mux3 : Mux  Inputs=3
  Switch : Switch  Criteria=u2 > Threshold  Threshold=75
  Wind Velocity : Outport
  wires:
  Constant7/1 -> Horizontal Wind Model 14/3
  Constant6/1 -> Horizontal Wind Model 14/2
  Mux3/1 -> Horizontal Wind Model 14/1
  height/1 -> Switch/2, Mux3/3
  Constant/1 -> Mux3/2
  Constant5/1 -> Mux3/1
  Horizontal Wind Model 14/1 -> Switch/1
  Switch/1 -> Wind Velocity/1
  Ground/1 -> Switch/3

== matlab function Purdue_Sim/Rocket/Animation Translation/MATLAB Function ==
  data: u input; y output
function y = fcn(u)
y = [0; 0; 0; 0];
y(1) = u(2)/sqrt(1-u(1)^2);
y(2) = u(3)/sqrt(1-u(1)^2);
y(3) = u(4)/sqrt(1-u(1)^2);
y(4) = 2 * acos(u(1));
end
